simulink model "rfi_sim_model"  (R2013b)
settings: Solver=ode45  StartTime=0.0  StopTime=37888  RelTol=1e-3
undefined symbols (not defined in the file or in its folder): calan_lib, comp_addsub
libraries: xbsIndex_r4 x886, casper_library_misc x64, xps_library x1
(part 1 of 9)
settings Model: Creator=root  LastModifiedBy=root

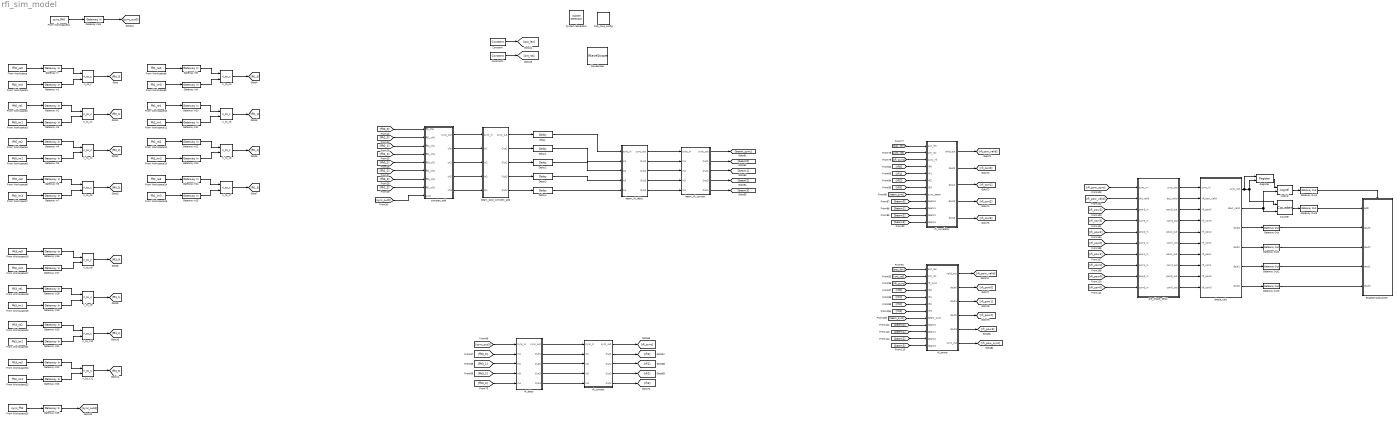
== system rfi_sim_model ==
  " System Generator" : xbsIndex_r4/ System Generator  Tag=genX  xilinxfamily=virtex6  part=xc6vsx475t  speed=-1  package=ff1759  synthesis_tool=XST  clock_wrapper=Clock Enables  directory=./arte/sysgen  proj_type=Project Navigator  Synth_file=XST Defaults  Impl_file=ISE Defaults  testbench=off  simulink_period=1  sysclk_period=6.6667  dcm_input_clock_period=100  incr_netlist=off  trim_vbits=Everywhere in SubSystem  dbl_ovrd=According to Block Masks  core_generation=According to Block Masks  run_coregen=off  deprecated_control=off  eval_field=0  block_type=sysgen
  Constant : xbsIndex_r4/Constant  const=64  gui_display_data_type=Fixed-point  arith_type=Unsigned  n_bits=16  bin_pt=0  preci_type=Single  exp_width=8  frac_width=24  explicit_period=on  period=1  equ=P=C  opselect=C  inp2=PCIN>>17  opr=+  inp1=P  carry=CIN  dbl_ovrd=off  block_type=constant
  Constant1 : xbsIndex_r4/Constant  const=0  gui_display_data_type=Boolean  arith_type=Boolean  n_bits=16  bin_pt=0  preci_type=Single  exp_width=8  frac_width=24  explicit_period=on  period=1  equ=P=C  opselect=C  inp2=PCIN>>17  opr=+  inp1=P  carry=CIN  dbl_ovrd=off  block_type=constant
  Counter : xbsIndex_r4/Counter  cnt_type=Free Running  cnt_to=Inf  operation=Up  start_count=0  cnt_by_val=1  arith_type=Unsigned  n_bits=9  bin_pt=0  load_pin=off  rst=on  en=on  explicit_period=on  period=1  dbl_ovrd=off  use_behavioral_HDL=off  implementation=Fabric  block_type=counter
  Delay{,1..4} (5 alike) : xbsIndex_r4/Delay  rst=off  infoeditControl=Selection of Reset will increase slice count due to use of real FFs and instead of SRLs  en=off  latency=1  dbl_ovrd=off  reg_retiming=off  block_type=delay
  Enabled Subsystem : Subsystem  TreatAsAtomicUnit=on
  From Workspace : FromWorkspace  VariableName=fft0_re0  SampleTime=1  Interpolate=off  OutputAfterFinalValue=Cyclic repetition
  From Workspace1 : FromWorkspace  VariableName=fft0_im0  SampleTime=1  Interpolate=off  OutputAfterFinalValue=Cyclic repetition
  From Workspace10 : FromWorkspace  VariableName=fft1_re1  SampleTime=1  Interpolate=off  OutputAfterFinalValue=Cyclic repetition
  From Workspace11 : FromWorkspace  VariableName=fft1_im1  SampleTime=1  Interpolate=off  OutputAfterFinalValue=Cyclic repetition
  From Workspace12 : FromWorkspace  VariableName=fft1_re2  SampleTime=1  Interpolate=off  OutputAfterFinalValue=Cyclic repetition
  From Workspace13 : FromWorkspace  VariableName=fft1_im2  SampleTime=1  Interpolate=off  OutputAfterFinalValue=Cyclic repetition
  From Workspace14 : FromWorkspace  VariableName=fft1_re3  SampleTime=1  Interpolate=off  OutputAfterFinalValue=Cyclic repetition
  From Workspace15 : FromWorkspace  VariableName=fft1_im3  SampleTime=1  Interpolate=off  OutputAfterFinalValue=Cyclic repetition
  From Workspace16 : FromWorkspace  VariableName=fft3_re0  SampleTime=1  Interpolate=off  OutputAfterFinalValue=Cyclic repetition
  From Workspace17 : FromWorkspace  VariableName=fft3_im0  SampleTime=1  Interpolate=off  OutputAfterFinalValue=Cyclic repetition
  From Workspace18 : FromWorkspace  VariableName=fft3_re1  SampleTime=1  Interpolate=off  OutputAfterFinalValue=Cyclic repetition
  From Workspace19 : FromWorkspace  VariableName=fft3_im1  SampleTime=1  Interpolate=off  OutputAfterFinalValue=Cyclic repetition
  From Workspace2 : FromWorkspace  VariableName=fft0_re1  SampleTime=1  Interpolate=off  OutputAfterFinalValue=Cyclic repetition
  From Workspace20 : FromWorkspace  VariableName=fft3_re2  SampleTime=1  Interpolate=off  OutputAfterFinalValue=Cyclic repetition
  From Workspace21 : FromWorkspace  VariableName=fft3_im2  SampleTime=1  Interpolate=off  OutputAfterFinalValue=Cyclic repetition
  From Workspace22 : FromWorkspace  VariableName=fft3_re3  SampleTime=1  Interpolate=off  OutputAfterFinalValue=Cyclic repetition
  From Workspace23 : FromWorkspace  VariableName=fft3_im3  SampleTime=1  Interpolate=off  OutputAfterFinalValue=Cyclic repetition
  From Workspace24 : FromWorkspace  VariableName=sync_fft0  SampleTime=1  Interpolate=off  OutputAfterFinalValue=Cyclic repetition
  From Workspace25 : FromWorkspace  VariableName=sync_fft3  SampleTime=1  Interpolate=off  OutputAfterFinalValue=Cyclic repetition
  From Workspace3 : FromWorkspace  VariableName=fft0_im1  SampleTime=1  Interpolate=off  OutputAfterFinalValue=Cyclic repetition
  From Workspace4 : FromWorkspace  VariableName=fft0_re2  SampleTime=1  Interpolate=off  OutputAfterFinalValue=Cyclic repetition
  From Workspace5 : FromWorkspace  VariableName=fft0_im2  SampleTime=1  Interpolate=off  OutputAfterFinalValue=Cyclic repetition
  From Workspace6 : FromWorkspace  VariableName=fft0_re3  SampleTime=1  Interpolate=off  OutputAfterFinalValue=Cyclic repetition
  From Workspace7 : FromWorkspace  VariableName=fft0_im3  SampleTime=1  Interpolate=off  OutputAfterFinalValue=Cyclic repetition
  From Workspace8 : FromWorkspace  VariableName=fft1_re0  SampleTime=1  Interpolate=off  OutputAfterFinalValue=Cyclic repetition
  From Workspace9 : FromWorkspace  VariableName=fft1_im0  SampleTime=1  Interpolate=off  OutputAfterFinalValue=Cyclic repetition
  Gateway In{,1..23} (24 alike) : xbsIndex_r4/Gateway In  gui_display_data_type=Fixed-point  arith_type="Signed  (2's comp)"  n_bits=18  bin_pt=17  preci_type=Single  exp_width=8  frac_width=24  quantization="Round  (unbiased: +/- Inf)"  overflow=Saturate  period=1  dbl_ovrd=off  timing_constraint=None  locs_specified=off  LOCs={}  UseAsADC=off  ADCChannel='1'  inherit_from_input=off  hdl_port=on  block_type=gatewayin
  Gateway In24 : xbsIndex_r4/Gateway In  gui_display_data_type=Boolean  arith_type=Boolean  n_bits=18  bin_pt=17  preci_type=Single  exp_width=8  frac_width=24  quantization="Round  (unbiased: +/- Inf)"  overflow=Saturate  period=1  dbl_ovrd=off  timing_constraint=None  locs_specified=off  LOCs={}  UseAsADC=off  ADCChannel='1'  inherit_from_input=off  hdl_port=on  block_type=gatewayin
  Gateway In25 : xbsIndex_r4/Gateway In  gui_display_data_type=Boolean  arith_type=Boolean  n_bits=18  bin_pt=17  preci_type=Single  exp_width=8  frac_width=24  quantization="Round  (unbiased: +/- Inf)"  overflow=Saturate  period=1  dbl_ovrd=off  timing_constraint=None  locs_specified=off  LOCs={}  UseAsADC=off  ADCChannel='1'  inherit_from_input=off  hdl_port=on  block_type=gatewayin
  Gateway Out{,1..5} (6 alike) : xbsIndex_r4/Gateway Out  inherit_from_input=off  hdl_port=on  timing_constraint=None  locs_specified=off  LOCs={}  UseAsDAC=off  DACChannel='1'  block_type=gatewayout
  Logical : xbsIndex_r4/Logical  logical_function=AND  inputs=2  en=off  latency=0  precision=Full  arith_type=Unsigned  n_bits=16  bin_pt=0  align_bp=on  dbl_ovrd=off  block_type=logical
  Register : xbsIndex_r4/Register  init=0  rst=off  en=on  dbl_ovrd=off  block_type=register
  WaveScope : xbsIndex_r4/WaveScope  block_type=wavescope
  XSG_core_config : xps_library/XSG_core_config  Tag=xps:xsg  hw_sys=ROACH2:sx475t  clk_src=adc0_clk  ROACH_clk_src=sys_clk  ROACH2_clk_src=adc0_clk  MKDIG_clk_src=sys_clk  clk_rate=150  sample_period=1  synthesis_tool=XST
  beam_post_complex_add : Subsystem  mask{lat=3}
  beam_rfi_convert : Subsystem  mask{shift_val=9, conv_width=9, conv_point=8}
      mask prompts: shift_val "shift"; conv_width "convert width"; conv_point "convert point"
  beam_rfi_delay : Subsystem  mask{lat=3}
  complex_add : Subsystem
  phase_calc : Subsystem  mask{din_width=16, din_point=2, scale_max_shift=10, scale_min_shift=3, pre_cordic_shift=0, pre_cordic_width=16, pre_cordic_point=2, cordic_iters=16}
      mask prompts: din_width "din width"; din_point "din point"; scale_max_shift "autoscale max shift"; scale_min_shift "autoscale min shift"; pre_cordic_shift "pre cordic shift"; pre_cordic_width "pre cordic width"; pre_cordic_point "pre cordic point"; cordic_iters "cordic iters"
  pre_phase_delay : Subsystem  mask{lat=2}
  rfi_convert : Subsystem  mask{shift_val=9, conv_width=9, conv_point=8}
      mask prompts: shift_val "shift"; conv_width "convert width"; conv_point "convert point"
  rfi_correlator : Subsystem  mask{din_width=9, din_point=8, cmult_width=18, cmult_point=16, cmult_add_dly=2, cmult_mult_dly=3, post_cmult_dly=1, acc_width=32, post_acc_dly=2, power_add_dly=2, power_mult_dly=3, dout_shift=11, dout_width=16, dout_point=2}
      mask prompts: din_width "din width"; din_point "din point"; cmult_width "cmult width"; cmult_point "cmult point"; cmult_add_dly "cmult add delay"; cmult_mult_dly "cmult mult delay"; post_cmult_dly "post cmult delay"; acc_width "acc width"; post_acc_dly "post acc delay"; power_add_dly "power add delay"; power_mult_dly "power mult delay"; dout_shift "output shift"; dout_width "output width"; dout_point "output point"
  rfi_delay : Subsystem  mask{lat=9}
  rfi_power : Subsystem  mask{din_width=9, din_point=8, pow_add_dly=2, pow_mult_dly=3, post_pow_dly=1, acc_width=32, post_acc_dly=2, post_acc_shift=0, post_acc_width=32, post_acc_point=16, cmult_add_dly=2, cmult_mult_dly=3, shift_out=11, dout_width=16, dout_point=2}
      mask prompts: din_width "din width"; pow_add_dly "power add delay"; pow_mult_dly "power mult delay"; post_pow_dly "post power delay"; acc_width "acc width"; post_acc_dly "post acc delay"; post_acc_shift "post acc shift"; post_acc_width "post acc width"; post_acc_point "post acc point"; cmult_add_dly "cmult add delay"; cmult_mult_dly "cmult mult delay"; shift_out "shift out"
  ri_to_c{,1..11} (12 alike) : casper_library_misc/ri_to_c
  wires:
  [fft0_0] -> complex_add/1(ff0_ch0)
  [fft1_0] -> complex_add/2(fft1_ch0)
  [fft0_1] -> complex_add/3(fft0_ch1)
  [fft1_1] -> complex_add/4(fft1_ch1)
  [fft0_2] -> complex_add/5(fft0_ch2)
  [fft1_2] -> complex_add/6(fft1_ch2)
  [fft0_3] -> complex_add/7(fft0_ch3)
  [fft1_3] -> complex_add/8(fft1_ch3)
  [sync_out0] -> complex_add/9(sync)
  complex_add/3(ch1) -> beam_post_complex_add/3(In2)
  complex_add/1(sync_out) -> beam_post_complex_add/1(sync_in)
  complex_add/2(ch0) -> beam_post_complex_add/2(In1)
  complex_add/5(ch3) -> beam_post_complex_add/5(In4)
  complex_add/4(ch2) -> beam_post_complex_add/4(In3)
  beam_post_complex_add/1(sync_out) -> Delay/1
  beam_post_complex_add/2(Out1) -> Delay1/1
  beam_post_complex_add/3(Out2) -> Delay2/1
  beam_post_complex_add/4(Out3) -> Delay3/1
  beam_post_complex_add/5(Out4) -> Delay4/1
  From Workspace/1 -> Gateway In/1
  From Workspace1/1 -> Gateway In1/1
  From Workspace2/1 -> Gateway In2/1
  From Workspace3/1 -> Gateway In3/1
  Gateway In/1 -> ri_to_c/1
  Gateway In1/1 -> ri_to_c/2
  Gateway In2/1 -> ri_to_c1/1
  Gateway In3/1 -> ri_to_c1/2
  From Workspace4/1 -> Gateway In4/1
  From Workspace5/1 -> Gateway In5/1
  From Workspace6/1 -> Gateway In6/1
  From Workspace7/1 -> Gateway In7/1
  Gateway In4/1 -> ri_to_c2/1
  Gateway In5/1 -> ri_to_c2/2
  Gateway In6/1 -> ri_to_c3/1
  Gateway In7/1 -> ri_to_c3/2
  ri_to_c/1 -> [fft0_0]
  ri_to_c1/1 -> [fft0_1]
  ri_to_c2/1 -> [fft0_2]
  ri_to_c3/1 -> [fft0_3]
  From Workspace8/1 -> Gateway In8/1
  From Workspace9/1 -> Gateway In9/1
  From Workspace10/1 -> Gateway In10/1
  From Workspace11/1 -> Gateway In11/1
  Gateway In8/1 -> ri_to_c4/1
  Gateway In9/1 -> ri_to_c4/2
  Gateway In10/1 -> ri_to_c5/1
  Gateway In11/1 -> ri_to_c5/2
  From Workspace12/1 -> Gateway In12/1
  From Workspace13/1 -> Gateway In13/1
  From Workspace14/1 -> Gateway In14/1
  From Workspace15/1 -> Gateway In15/1
  Gateway In12/1 -> ri_to_c6/1
  Gateway In13/1 -> ri_to_c6/2
  Gateway In14/1 -> ri_to_c7/1
  Gateway In15/1 -> ri_to_c7/2
  ri_to_c4/1 -> [fft1_0]
  ri_to_c5/1 -> [fft1_1]
  ri_to_c6/1 -> [fft1_2]
  ri_to_c7/1 -> [fft1_3]
  From Workspace16/1 -> Gateway In16/1
  From Workspace17/1 -> Gateway In17/1
  From Workspace18/1 -> Gateway In18/1
  From Workspace19/1 -> Gateway In19/1
  Gateway In16/1 -> ri_to_c8/1
  Gateway In17/1 -> ri_to_c8/2
  Gateway In18/1 -> ri_to_c9/1
  Gateway In19/1 -> ri_to_c9/2
  From Workspace20/1 -> Gateway In20/1
  From Workspace21/1 -> Gateway In21/1
  From Workspace22/1 -> Gateway In22/1
  From Workspace23/1 -> Gateway In23/1
  Gateway In20/1 -> ri_to_c10/1
  Gateway In21/1 -> ri_to_c10/2
  Gateway In22/1 -> ri_to_c11/1
  Gateway In23/1 -> ri_to_c11/2
  ri_to_c8/1 -> [fft3_0]
  ri_to_c9/1 -> [fft3_1]
  ri_to_c10/1 -> [fft3_2]
  ri_to_c11/1 -> [fft3_3]
  From Workspace24/1 -> Gateway In24/1
  Gateway In24/1 -> [sync_out0]
  From Workspace25/1 -> Gateway In25/1
  Gateway In25/1 -> [sync_out3]
  Delay/1 -> beam_rfi_delay/1(sync_in)
  Delay1/1 -> beam_rfi_delay/2(In1)
  Delay2/1 -> beam_rfi_delay/3(In2)
  Delay3/1 -> beam_rfi_delay/4(In3)
  Delay4/1 -> beam_rfi_delay/5(In4)
  Constant/1 -> [acc_len]
  Constant1/1 -> [cnt_rst]
  [acc_len] -> rfi_correlator/1(acc_len)
  [cnt_rst] -> rfi_correlator/2(cnt_rst)
  [rfi_sync] -> rfi_correlator/3(sync_rfi)
  [rfi0] -> rfi_correlator/4(rfi0)
  [rfi1] -> rfi_correlator/5(rfi1)
  [rfi2] -> rfi_correlator/6(rfi2)
  [rfi3] -> rfi_correlator/7(rfi3)
  [beam_sync] -> rfi_correlator/8(sync_beam)
  [beam0] -> rfi_correlator/9(beam0)
  [beam1] -> rfi_correlator/10(beam1)
  [beam2] -> rfi_correlator/11(beam2)
  [beam3] -> rfi_correlator/12(beam3)
  [acc_len] -> rfi_power/1(acc_len)
  [cnt_rst] -> rfi_power/2(cnt_rst)
  [rfi_sync] -> rfi_power/3(rfi_sync)
  [rfi0] -> rfi_power/4(rfi0)
  [rfi1] -> rfi_power/5(rfi1)
  [rfi2] -> rfi_power/6(rfi2)
  [rfi3] -> rfi_power/7(rfi3)
  [beam_sync] -> rfi_power/8(beam_sync)
  [beam0] -> rfi_power/9(beam0)
  [beam1] -> rfi_power/10(beam1)
  [beam2] -> rfi_power/11(beam2)
  [beam3] -> rfi_power/12(beam3)
  rfi_correlator/1(valid_out) -> [rfi_corr_valid]
  rfi_correlator/2(dout0) -> [rfi_corr0]
  rfi_correlator/3(dout1) -> [rfi_corr1]
  rfi_correlator/4(dout2) -> [rfi_corr2]
  rfi_correlator/5(dout3) -> [rfi_corr3]
  rfi_power/1(valid_out) -> [rfi_pow_valid]
  rfi_power/2(dout0) -> [rfi_pow0]
  rfi_power/3(dout1) -> [rfi_pow1]
  rfi_power/4(dout2) -> [rfi_pow2]
  rfi_power/5(dout3) -> [rfi_pow3]
  rfi_power/6(sync_out) -> [rfi_pow_sync]
  pre_phase_delay/3(pow3_out) -> phase_calc/3(rfi_pow3)
  pre_phase_delay/9(pow0_out) -> phase_calc/9(rfi_pow0)
  pre_phase_delay/5(pow2_out) -> phase_calc/5(rfi_pow2)
  pre_phase_delay/8(corr1_out) -> phase_calc/8(rfi_corr1)
  pre_phase_delay/1(sync_out) -> phase_calc/1(sync_in)
  pre_phase_delay/6(corr2_out) -> phase_calc/6(rfi_corr2)
  pre_phase_delay/10(corr0_out) -> phase_calc/10(rfi_corr0)
  pre_phase_delay/4(corr3_out) -> phase_calc/4(rfi_corr3)
  pre_phase_delay/7(pow1_out) -> phase_calc/7(rfi_pow1)
  pre_phase_delay/2(dou_valid) -> phase_calc/2(rfi_pow_valid)
  [rfi_pow_sync] -> pre_phase_delay/1(sync_in)
  [rfi_pow_valid] -> pre_phase_delay/2(din_valid)
  [rfi_pow3] -> pre_phase_delay/3(pow3_in)
  [rfi_corr3] -> pre_phase_delay/4(corr3_in)
  [rfi_pow2] -> pre_phase_delay/5(pow2_in)
  [rfi_corr2] -> pre_phase_delay/6(corr2_in)
  [rfi_pow1] -> pre_phase_delay/7(pow1_in)
  [rfi_corr1] -> pre_phase_delay/8(corr1_in)
  [rfi_pow0] -> pre_phase_delay/9(pow0_in)
  [rfi_corr0] -> pre_phase_delay/10(corr0_in)
  rfi_delay/2(Out1) -> rfi_convert/2(In1)
  rfi_delay/3(Out2) -> rfi_convert/3(In2)
  rfi_delay/1(sync_out) -> rfi_convert/1(sync_in)
  rfi_delay/4(Out3) -> rfi_convert/4(In3)
  rfi_delay/5(Out4) -> rfi_convert/5(In4)
  [sync_out3] -> rfi_delay/1(sync_in)
  [fft3_0] -> rfi_delay/2(In1)
  [fft3_1] -> rfi_delay/3(In2)
  [fft3_2] -> rfi_delay/4(In3)
  [fft3_3] -> rfi_delay/5(In4)
  rfi_convert/1(sync_out) -> [rfi_sync]
  rfi_convert/2(Out1) -> [rfi0]
  rfi_convert/3(Out2) -> [rfi1]
  rfi_convert/4(Out3) -> [rfi2]
  rfi_convert/5(Out4) -> [rfi3]
  beam_rfi_delay/2(Out1) -> beam_rfi_convert/2(In1)
  beam_rfi_delay/3(Out2) -> beam_rfi_convert/3(In2)
  beam_rfi_delay/1(sync_out) -> beam_rfi_convert/1(sync_in)
  beam_rfi_delay/4(Out3) -> beam_rfi_convert/4(In3)
  beam_rfi_delay/5(Out4) -> beam_rfi_convert/5(In4)
  beam_rfi_convert/1(sync_out) -> [beam_sync]
  beam_rfi_convert/2(Out1) -> [beam0]
  beam_rfi_convert/3(Out2) -> [beam1]
  beam_rfi_convert/4(Out3) -> [beam2]
  beam_rfi_convert/5(Out4) -> [beam3]
  phase_calc/3(dout3) -> Gateway Out/1
  phase_calc/4(dout2) -> Gateway Out1/1
  phase_calc/5(dout1) -> Gateway Out2/1
  phase_calc/6(dout0) -> Gateway Out3/1
  phase_calc/1(sync_out) -> Register/1, Counter/1, Register/2
  phase_calc/2(dout_valid) -> Logical/2, Counter/2
  Register/1 -> Logical/1
  Logical/1 -> Gateway Out4/1
  Gateway Out4/1 -> Enabled Subsystem/Enable
  Gateway Out/1 -> Enabled Subsystem/2(dout3)
  Gateway Out1/1 -> Enabled Subsystem/3(dout2)
  Gateway Out2/1 -> Enabled Subsystem/4(dout1)
  Gateway Out3/1 -> Enabled Subsystem/5(dout0)
  Counter/1 -> Gateway Out5/1
  Gateway Out5/1 -> Enabled Subsystem/1(addr)

== system rfi_sim_model/Enabled Subsystem ==
  addr : Inport
  dout3 : Inport  Port=2
  dout2 : Inport  Port=3
  dout1 : Inport  Port=4
  dout0 : Inport  Port=5
  Enable : EnablePort
  To Workspace : ToWorkspace  VariableName=dout3  SampleTime=-1  SaveFormat=Timeseries
  To Workspace1 : ToWorkspace  VariableName=dout2  SampleTime=-1  SaveFormat=Timeseries
  To Workspace2 : ToWorkspace  VariableName=dout1  SampleTime=-1  SaveFormat=Timeseries
  To Workspace3 : ToWorkspace  VariableName=dout0  SampleTime=-1  SaveFormat=Timeseries
  To Workspace4 : ToWorkspace  VariableName=addr  SampleTime=-1  SaveFormat=Timeseries
  wires:
  dout3/1 -> To Workspace/1
  dout2/1 -> To Workspace1/1
  dout1/1 -> To Workspace2/1
  dout0/1 -> To Workspace3/1
  addr/1 -> To Workspace4/1

== system rfi_sim_model/beam_post_complex_add ==
  sync_in : Inport
  In1 : Inport  Port=2
  In2 : Inport  Port=3
  In3 : Inport  Port=4
  In4 : Inport  Port=5
  pipeline1 : Subsystem  AncestorBlock=casper_library_delays/pipeline  mask(pipeline){latency=lat}
      mask help:
      | An explicitly laid-out delay line to avoid mapping to SRL16s
      | for use in pipelining to help achieve timing closure.
      mask init:
      | pipeline_init(gcb,'latency',latency);
      settings: AttributesFormatString=Latency = %<latency>
      mask Display:
      | port_label('input', 1, 'd');
      | port_label('output', 1, 'q');
      | disp(['Z^-', num2str(latency)]);
  pipeline2 : Subsystem  AncestorBlock=casper_library_delays/pipeline  mask(pipeline){latency=lat}
      mask help:
      | An explicitly laid-out delay line to avoid mapping to SRL16s
      | for use in pipelining to help achieve timing closure.
      mask init:
      | pipeline_init(gcb,'latency',latency);
      settings: AttributesFormatString=Latency = %<latency>
      mask Display:
      | port_label('input', 1, 'd');
      | port_label('output', 1, 'q');
      | disp(['Z^-', num2str(latency)]);
  pipeline3 : Subsystem  AncestorBlock=casper_library_delays/pipeline  mask(pipeline){latency=lat}
      mask help:
      | An explicitly laid-out delay line to avoid mapping to SRL16s
      | for use in pipelining to help achieve timing closure.
      mask init:
      | pipeline_init(gcb,'latency',latency);
      settings: AttributesFormatString=Latency = %<latency>
      mask Display:
      | port_label('input', 1, 'd');
      | port_label('output', 1, 'q');
      | disp(['Z^-', num2str(latency)]);
  pipeline4 : Subsystem  AncestorBlock=casper_library_delays/pipeline  mask(pipeline){latency=lat}
      mask help:
      | An explicitly laid-out delay line to avoid mapping to SRL16s
      | for use in pipelining to help achieve timing closure.
      mask init:
      | pipeline_init(gcb,'latency',latency);
      settings: AttributesFormatString=Latency = %<latency>
      mask Display:
      | port_label('input', 1, 'd');
      | port_label('output', 1, 'q');
      | disp(['Z^-', num2str(latency)]);
  pipeline5 : Subsystem  AncestorBlock=casper_library_delays/pipeline  mask(pipeline){latency=lat}
      mask help:
      | An explicitly laid-out delay line to avoid mapping to SRL16s
      | for use in pipelining to help achieve timing closure.
      mask init:
      | pipeline_init(gcb,'latency',latency);
      settings: AttributesFormatString=Latency = %<latency>
      mask Display:
      | port_label('input', 1, 'd');
      | port_label('output', 1, 'q');
      | disp(['Z^-', num2str(latency)]);
  sync_out : Outport
  Out1 : Outport  Port=2
  Out2 : Outport  Port=3
  Out3 : Outport  Port=4
  Out4 : Outport  Port=5
  wires:
  sync_in/1 -> pipeline1/1(d)
  pipeline1/1(q) -> sync_out/1
  In1/1 -> pipeline2/1(d)
  pipeline2/1(q) -> Out1/1
  In2/1 -> pipeline3/1(d)
  pipeline3/1(q) -> Out2/1
  In3/1 -> pipeline4/1(d)
  pipeline4/1(q) -> Out3/1
  In4/1 -> pipeline5/1(d)
  pipeline5/1(q) -> Out4/1

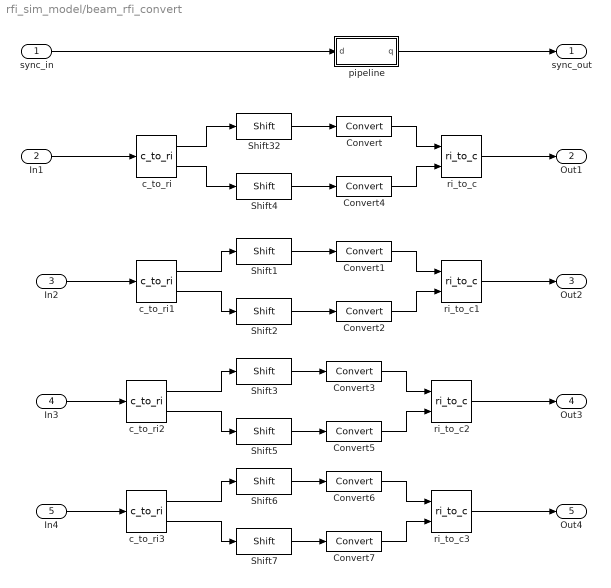
== system rfi_sim_model/beam_rfi_convert ==
  sync_in : Inport
  In1 : Inport  Port=2
  In2 : Inport  Port=3
  In3 : Inport  Port=4
  In4 : Inport  Port=5
  Convert{,1..7} (8 alike) : xbsIndex_r4/Convert  gui_display_data_type=Fixed-point  arith_type="Signed  (2's comp)"  n_bits=conv_width  bin_pt=conv_point  float_type=Single  exp_bits=8  fraction_bits=24  quantization=Truncate  overflow=Wrap  en=off  latency=2  dbl_ovrd=off  pipeline=off  block_type=convert
      settings: block_version=11.4
  Shift{1..7,32} (8 alike) : xbsIndex_r4/Shift  shift_dir=Left  shift_bits=shift_val  en=off  latency=0  precision=Full  arith_type="Signed  (2's comp)"  n_bits=16  bin_pt=14  quantization=Truncate  overflow=Wrap  dbl_ovrd=off  block_type=shift
  c_to_ri{,1..3} (4 alike) : casper_library_misc/c_to_ri  n_bits=18  bin_pt=17
  pipeline : Subsystem  AncestorBlock=casper_library_delays/pipeline  mask(pipeline){latency=2}
      mask help:
      | An explicitly laid-out delay line to avoid mapping to SRL16s
      | for use in pipelining to help achieve timing closure.
      mask init:
      | pipeline_init(gcb,'latency',latency);
      settings: AttributesFormatString=Latency = %<latency>
      mask Display:
      | port_label('input', 1, 'd');
      | port_label('output', 1, 'q');
      | disp(['Z^-', num2str(latency)]);
  ri_to_c{,1..3} (4 alike) : casper_library_misc/ri_to_c
  sync_out : Outport
  Out1 : Outport  Port=2
  Out2 : Outport  Port=3
  Out3 : Outport  Port=4
  Out4 : Outport  Port=5
  wires:
  Shift32/1 -> Convert/1
  sync_in/1 -> pipeline/1(d)
  pipeline/1(q) -> sync_out/1
  In1/1 -> c_to_ri/1
  c_to_ri/1 -> Shift32/1
  ri_to_c/1 -> Out1/1
  Convert/1 -> ri_to_c/1
  Shift4/1 -> Convert4/1
  c_to_ri/2 -> Shift4/1
  Convert4/1 -> ri_to_c/2
  Shift1/1 -> Convert1/1
  c_to_ri1/1 -> Shift1/1
  ri_to_c1/1 -> Out2/1
  Convert1/1 -> ri_to_c1/1
  Shift2/1 -> Convert2/1
  c_to_ri1/2 -> Shift2/1
  Convert2/1 -> ri_to_c1/2
  In2/1 -> c_to_ri1/1
  Shift3/1 -> Convert3/1
  c_to_ri2/1 -> Shift3/1
  ri_to_c2/1 -> Out3/1
  Convert3/1 -> ri_to_c2/1
  Shift5/1 -> Convert5/1
  c_to_ri2/2 -> Shift5/1
  Convert5/1 -> ri_to_c2/2
  In3/1 -> c_to_ri2/1
  Shift6/1 -> Convert6/1
  c_to_ri3/1 -> Shift6/1
  ri_to_c3/1 -> Out4/1
  Convert6/1 -> ri_to_c3/1
  Shift7/1 -> Convert7/1
  c_to_ri3/2 -> Shift7/1
  Convert7/1 -> ri_to_c3/2
  In4/1 -> c_to_ri3/1

== system rfi_sim_model/beam_rfi_delay ==
  sync_in : Inport
  In1 : Inport  Port=2
  In2 : Inport  Port=3
  In3 : Inport  Port=4
  In4 : Inport  Port=5
  pipeline1 : Subsystem  AncestorBlock=casper_library_delays/pipeline  mask(pipeline){latency=lat}
      mask help:
      | An explicitly laid-out delay line to avoid mapping to SRL16s
      | for use in pipelining to help achieve timing closure.
      mask init:
      | pipeline_init(gcb,'latency',latency);
      settings: AttributesFormatString=Latency = %<latency>
      mask Display:
      | port_label('input', 1, 'd');
      | port_label('output', 1, 'q');
      | disp(['Z^-', num2str(latency)]);
  pipeline2 : Subsystem  AncestorBlock=casper_library_delays/pipeline  mask(pipeline){latency=lat}
      mask help:
      | An explicitly laid-out delay line to avoid mapping to SRL16s
      | for use in pipelining to help achieve timing closure.
      mask init:
      | pipeline_init(gcb,'latency',latency);
      settings: AttributesFormatString=Latency = %<latency>
      mask Display:
      | port_label('input', 1, 'd');
      | port_label('output', 1, 'q');
      | disp(['Z^-', num2str(latency)]);
  pipeline3 : Subsystem  AncestorBlock=casper_library_delays/pipeline  mask(pipeline){latency=lat}
      mask help:
      | An explicitly laid-out delay line to avoid mapping to SRL16s
      | for use in pipelining to help achieve timing closure.
      mask init:
      | pipeline_init(gcb,'latency',latency);
      settings: AttributesFormatString=Latency = %<latency>
      mask Display:
      | port_label('input', 1, 'd');
      | port_label('output', 1, 'q');
      | disp(['Z^-', num2str(latency)]);
  pipeline4 : Subsystem  AncestorBlock=casper_library_delays/pipeline  mask(pipeline){latency=lat}
      mask help:
      | An explicitly laid-out delay line to avoid mapping to SRL16s
      | for use in pipelining to help achieve timing closure.
      mask init:
      | pipeline_init(gcb,'latency',latency);
      settings: AttributesFormatString=Latency = %<latency>
      mask Display:
      | port_label('input', 1, 'd');
      | port_label('output', 1, 'q');
      | disp(['Z^-', num2str(latency)]);
  pipeline5 : Subsystem  AncestorBlock=casper_library_delays/pipeline  mask(pipeline){latency=lat}
      mask help:
      | An explicitly laid-out delay line to avoid mapping to SRL16s
      | for use in pipelining to help achieve timing closure.
      mask init:
      | pipeline_init(gcb,'latency',latency);
      settings: AttributesFormatString=Latency = %<latency>
      mask Display:
      | port_label('input', 1, 'd');
      | port_label('output', 1, 'q');
      | disp(['Z^-', num2str(latency)]);
  sync_out : Outport
  Out1 : Outport  Port=2
  Out2 : Outport  Port=3
  Out3 : Outport  Port=4
  Out4 : Outport  Port=5
  wires:
  sync_in/1 -> pipeline1/1(d)
  pipeline1/1(q) -> sync_out/1
  In1/1 -> pipeline2/1(d)
  pipeline2/1(q) -> Out1/1
  In2/1 -> pipeline3/1(d)
  pipeline3/1(q) -> Out2/1
  In3/1 -> pipeline4/1(d)
  pipeline4/1(q) -> Out3/1
  In4/1 -> pipeline5/1(d)
  pipeline5/1(q) -> Out4/1

== system rfi_sim_model/complex_add ==
  ff0_ch0 : Inport
  fft1_ch0 : Inport  Port=2
  fft0_ch1 : Inport  Port=3
  fft1_ch1 : Inport  Port=4
  fft0_ch2 : Inport  Port=5
  fft1_ch2 : Inport  Port=6
  fft0_ch3 : Inport  Port=7
  fft1_ch3 : Inport  Port=8
  sync : Inport  Port=9
  comp_addsub : Subsystem  AncestorBlock=calan_lib/comp_addsub  mask(comp_addsub){addsub=Addition, n_bits_in=18, bin_pt_in=17, add_latency=2, n_bits_out=18, bin_pt_out=17, quantization=Truncate, overflow=Wrap}
      mask prompts: addsub "Addition/Subtraction"; n_bits_in "Bit Width"; bin_pt_in "Binary Point"; add_latency "Adder Latency"; n_bits_out "Bit Width"; bin_pt_out "BInary Point"
      mask help: Add or substract two complex numbers of the same length.
      mask init:
      | comp_addsub_init(gcb, ...
      |     'addsub', addsub, ...
      |     'n_bits_in', n_bits_in, ...
      |     'bin_pt_in', bin_pt_in, ...
      |     'n_bits_out', n_bits_out, ...
      |     'bin_pt_out', bin_pt_out, ...
      |     'quantization', quantization, ...
      |     'overflow', overflow, ...
      |     'add_latency', add_latency);
      settings: AttributesFormatString=|
      | 18_17 * 18_17 ==> 18_17
      | Truncate, Wrap
      mask TypeOptions addsub: Addition | Subtraction
      mask TypeOptions quantization: Truncate | Round  (unbiased: +/- Inf)
      mask TypeOptions overflow: Wrap | Saturate | Flag as error
      mask Display:
      | port_label('input', 1, 'a');
      | port_label('input', 2, 'b');
      | if strcmp(addsub, 'Addition')
      |     port_label('output', 1, 'a+b');
      | elseif strcmp(addsub, 'Subtraction')
      |     port_label('output', 1, 'a-b');
      | end
      | disp(['Z^-', num2str(add_latency)]);
  comp_addsub1 : Subsystem  AncestorBlock=calan_lib/comp_addsub  mask(comp_addsub){addsub=Addition, n_bits_in=18, bin_pt_in=17, add_latency=2, n_bits_out=18, bin_pt_out=17, quantization=Truncate, overflow=Wrap}
      mask prompts: addsub "Addition/Subtraction"; n_bits_in "Bit Width"; bin_pt_in "Binary Point"; add_latency "Adder Latency"; n_bits_out "Bit Width"; bin_pt_out "BInary Point"
      mask help: Add or substract two complex numbers of the same length.
      mask init: same as rfi_sim_model/complex_add/comp_addsub
      settings: AttributesFormatString=|
      | 18_17 * 18_17 ==> 18_17
      | Truncate, Wrap
      mask TypeOptions addsub: Addition | Subtraction
      mask TypeOptions quantization: Truncate | Round  (unbiased: +/- Inf)
      mask TypeOptions overflow: Wrap | Saturate | Flag as error
      mask Display:
      | port_label('input', 1, 'a');
      | port_label('input', 2, 'b');
      | if strcmp(addsub, 'Addition')
      |     port_label('output', 1, 'a+b');
      | elseif strcmp(addsub, 'Subtraction')
      |     port_label('output', 1, 'a-b');
      | end
      | disp(['Z^-', num2str(add_latency)]);
  comp_addsub3 : Subsystem  AncestorBlock=calan_lib/comp_addsub  mask(comp_addsub){addsub=Addition, n_bits_in=18, bin_pt_in=17, add_latency=2, n_bits_out=18, bin_pt_out=17, quantization=Truncate, overflow=Wrap}
      mask prompts: addsub "Addition/Subtraction"; n_bits_in "Bit Width"; bin_pt_in "Binary Point"; add_latency "Adder Latency"; n_bits_out "Bit Width"; bin_pt_out "BInary Point"
      mask help: Add or substract two complex numbers of the same length.
      mask init: same as rfi_sim_model/complex_add/comp_addsub
      settings: AttributesFormatString=|
      | 18_17 * 18_17 ==> 18_17
      | Truncate, Wrap
      mask TypeOptions addsub: Addition | Subtraction
      mask TypeOptions quantization: Truncate | Round  (unbiased: +/- Inf)
      mask TypeOptions overflow: Wrap | Saturate | Flag as error
      mask Display:
      | port_label('input', 1, 'a');
      | port_label('input', 2, 'b');
      | if strcmp(addsub, 'Addition')
      |     port_label('output', 1, 'a+b');
      | elseif strcmp(addsub, 'Subtraction')
      |     port_label('output', 1, 'a-b');
      | end
      | disp(['Z^-', num2str(add_latency)]);
  comp_addsub6 : Subsystem  AncestorBlock=calan_lib/comp_addsub  mask(comp_addsub){addsub=Addition, n_bits_in=18, bin_pt_in=17, add_latency=2, n_bits_out=18, bin_pt_out=17, quantization=Truncate, overflow=Wrap}
      mask prompts: addsub "Addition/Subtraction"; n_bits_in "Bit Width"; bin_pt_in "Binary Point"; add_latency "Adder Latency"; n_bits_out "Bit Width"; bin_pt_out "BInary Point"
      mask help: Add or substract two complex numbers of the same length.
      mask init: same as rfi_sim_model/complex_add/comp_addsub
      settings: AttributesFormatString=|
      | 18_17 * 18_17 ==> 18_17
      | Truncate, Wrap
      mask TypeOptions addsub: Addition | Subtraction
      mask TypeOptions quantization: Truncate | Round  (unbiased: +/- Inf)
      mask TypeOptions overflow: Wrap | Saturate | Flag as error
      mask Display:
      | port_label('input', 1, 'a');
      | port_label('input', 2, 'b');
      | if strcmp(addsub, 'Addition')
      |     port_label('output', 1, 'a+b');
      | elseif strcmp(addsub, 'Subtraction')
      |     port_label('output', 1, 'a-b');
      | end
      | disp(['Z^-', num2str(add_latency)]);
  pipeline4 : Subsystem  AncestorBlock=casper_library_delays/pipeline  mask(pipeline){latency=2}
      mask help:
      | An explicitly laid-out delay line to avoid mapping to SRL16s
      | for use in pipelining to help achieve timing closure.
      mask init:
      | pipeline_init(gcb,'latency',latency);
      settings: AttributesFormatString=Latency = %<latency>
      mask Display:
      | port_label('input', 1, 'd');
      | port_label('output', 1, 'q');
      | disp(['Z^-', num2str(latency)]);
  sync_out : Outport
  ch0 : Outport  Port=2
  ch1 : Outport  Port=3
  ch2 : Outport  Port=4
  ch3 : Outport  Port=5
  wires:
  ff0_ch0/1 -> comp_addsub/1(a)
  fft1_ch0/1 -> comp_addsub/2(b)
  fft0_ch1/1 -> comp_addsub1/1(a)
  fft1_ch1/1 -> comp_addsub1/2(b)
  fft0_ch2/1 -> comp_addsub3/1(a)
  comp_addsub3/1(out) -> ch2/1
  fft1_ch2/1 -> comp_addsub3/2(b)
  fft0_ch3/1 -> comp_addsub6/1(a)
  fft1_ch3/1 -> comp_addsub6/2(b)
  sync/1 -> pipeline4/1(d)
  pipeline4/1(q) -> sync_out/1
  comp_addsub/1(out) -> ch0/1
  comp_addsub6/1(out) -> ch3/1
  comp_addsub1/1(out) -> ch1/1

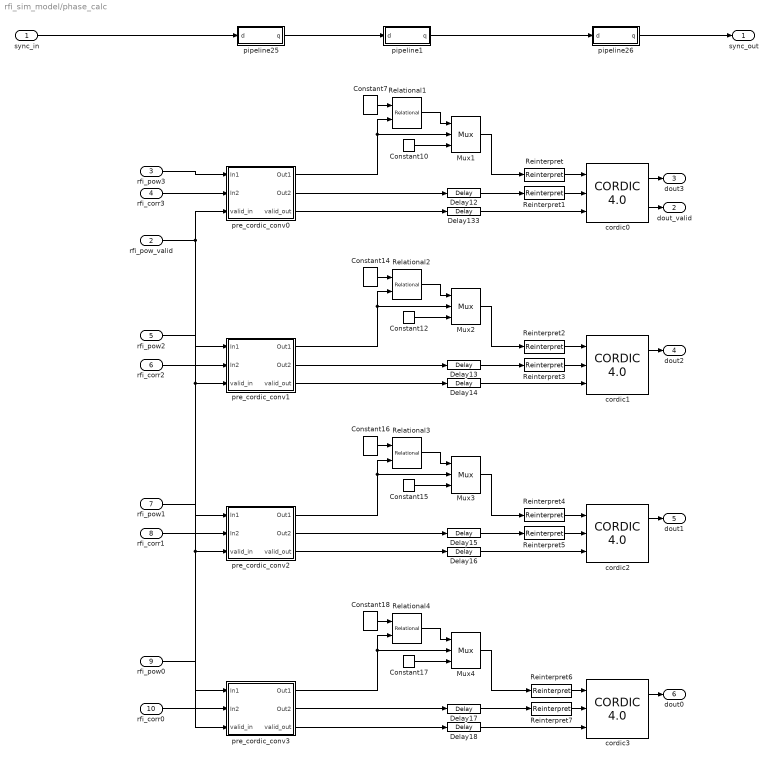
== system rfi_sim_model/phase_calc ==
  sync_in : Inport
  rfi_pow_valid : Inport  Port=2
  rfi_pow3 : Inport  Port=3
  rfi_corr3 : Inport  Port=4
  rfi_pow2 : Inport  Port=5
  rfi_corr2 : Inport  Port=6
  rfi_pow1 : Inport  Port=7
  rfi_corr1 : Inport  Port=8
  rfi_pow0 : Inport  Port=9
  rfi_corr0 : Inport  Port=10
  Constant{10,12,15,17} (4 alike) : xbsIndex_r4/Constant  const=1  gui_display_data_type=Fixed-point  arith_type=Signed (2's comp)  n_bits=pre_cordic_width  bin_pt=pre_cordic_point  preci_type=Single  exp_width=8  frac_width=24  explicit_period=on  period=1  equ=P=C  opselect=C  inp2=PCIN>>17  opr=+  inp1=P  carry=CIN  dbl_ovrd=off  block_type=constant
  Constant{7,14,16,18} (4 alike) : xbsIndex_r4/Constant  const=0  gui_display_data_type=Fixed-point  arith_type=Signed (2's comp)  n_bits=pre_cordic_width  bin_pt=pre_cordic_point  preci_type=Single  exp_width=8  frac_width=24  explicit_period=on  period=1  equ=P=C  opselect=C  inp2=PCIN>>17  opr=+  inp1=P  carry=CIN  dbl_ovrd=off  block_type=constant
  Delay{12..18,133} (8 alike) : xbsIndex_r4/Delay  rst=off  infoeditControl=Selection of Reset will increase slice count due to use of real FFs and instead of SRLs  en=off  latency=1  dbl_ovrd=off  reg_retiming=off  block_type=delay
  Mux{1..4} (4 alike) : xbsIndex_r4/Mux  inputs=2  en=off  latency=1  precision=Full  arith_type=Unsigned  n_bits=16  bin_pt=14  quantization=Truncate  overflow=Wrap  dbl_ovrd=off  block_type=mux
  Reinterpret{,1..7} (8 alike) : xbsIndex_r4/Reinterpret  force_arith_type=off  arith_type=Unsigned  force_bin_pt=on  bin_pt=pre_cordic_width-2  block_type=reinterpret
  Relational{1..4} (4 alike) : xbsIndex_r4/Relational  mode=a=b  en=off  latency=0  dbl_ovrd=off  block_type=relational
  cordic{0..3} (4 alike) : xbsIndex_r4/CORDIC 4.0   functional_selection=Arc_Tan  architectural_configuration=Parallel  pipelining_mode=Maximum  data_format=SignedFraction  phase_format=Radians  output_width=cordic_iters  round_mode=Truncate  iterations=cordic_iters  precision=0  coarse_rotation=off  compensation_scaling=No_Scale_Compensation  ce=off  sclr=off  nd=on  rdy=on  x_out=off  y_out=off  phase_output=on  register_inputs=true  register_outputs=true  ipcore_usecache=true  ipcore_useipmodelcache=true  ipcore_verbose=false  wrapper_available=true  ip_name=CORDIC  ip_version=4.0  dsptool_ready=true  port_translation_map={ 'ce' => 'en', 'sclr' => 'rst' }  structural_sim=false  block_type=cordic_v4_0
  pipeline1 : Subsystem  AncestorBlock=casper_library_delays/pipeline  mask(pipeline){latency=1}
      mask help:
      | An explicitly laid-out delay line to avoid mapping to SRL16s
      | for use in pipelining to help achieve timing closure.
      mask init:
      | pipeline_init(gcb,'latency',latency);
      settings: AttributesFormatString=Latency = %<latency>
      mask Display:
      | port_label('input', 1, 'd');
      | port_label('output', 1, 'q');
      | disp(['Z^-', num2str(latency)]);
  pipeline25 : Subsystem  AncestorBlock=casper_library_delays/pipeline  mask(pipeline){latency=2}
      mask help:
      | An explicitly laid-out delay line to avoid mapping to SRL16s
      | for use in pipelining to help achieve timing closure.
      mask init:
      | pipeline_init(gcb,'latency',latency);
      settings: AttributesFormatString=Latency = %<latency>
      mask Display:
      | port_label('input', 1, 'd');
      | port_label('output', 1, 'q');
      | disp(['Z^-', num2str(latency)]);
  pipeline26 : Subsystem  AncestorBlock=casper_library_delays/pipeline  mask(pipeline){latency=cordic_iters+2}
      mask help:
      | An explicitly laid-out delay line to avoid mapping to SRL16s
      | for use in pipelining to help achieve timing closure.
      mask init:
      | pipeline_init(gcb,'latency',latency);
      settings: AttributesFormatString=Latency = %<latency>
      mask Display:
      | port_label('input', 1, 'd');
      | port_label('output', 1, 'q');
      | disp(['Z^-', num2str(latency)]);
  pre_cordic_conv0 : Subsystem  mask{shift_val=pre_cordic_shift, conv_width=pre_cordic_width, conv_point=pre_cordic_point}
      mask prompts: shift_val "shift"; conv_width "convert width"; conv_point "convert point"
  pre_cordic_conv1 : Subsystem  mask{shift_val=pre_cordic_shift, conv_width=pre_cordic_width, conv_point=pre_cordic_point}
      mask prompts: shift_val "shift"; conv_width "convert width"; conv_point "convert point"
  pre_cordic_conv2 : Subsystem  mask{shift_val=pre_cordic_shift, conv_width=pre_cordic_width, conv_point=pre_cordic_point}
      mask prompts: shift_val "shift"; conv_width "convert width"; conv_point "convert point"
  pre_cordic_conv3 : Subsystem  mask{shift_val=pre_cordic_shift, conv_width=pre_cordic_width, conv_point=pre_cordic_point}
      mask prompts: shift_val "shift"; conv_width "convert width"; conv_point "convert point"
  sync_out : Outport
  dout_valid : Outport  Port=2
  dout3 : Outport  Port=3
  dout2 : Outport  Port=4
  dout1 : Outport  Port=5
  dout0 : Outport  Port=6
  wires:
  rfi_pow1/1 -> pre_cordic_conv2/1(In1)
  Delay14/1 -> cordic1/3
  pre_cordic_conv2/2(Out2) -> Delay15/1
  Mux3/1 -> Reinterpret4/1
  cordic1/1 -> dout2/1
  pipeline26/1(q) -> sync_out/1
  Delay13/1 -> Reinterpret3/1
  pre_cordic_conv1/2(Out2) -> Delay13/1
  Mux2/1 -> Reinterpret2/1
  pre_cordic_conv1/3(valid_out) -> Delay14/1
  Constant15/1 -> Mux3/3
  Delay15/1 -> Reinterpret5/1
  cordic0/2 -> dout_valid/1
  Constant16/1 -> Relational3/1
  rfi_corr1/1 -> pre_cordic_conv2/2(In2)
  rfi_pow0/1 -> pre_cordic_conv3/1(In1)
  rfi_corr0/1 -> pre_cordic_conv3/2(In2)
  rfi_pow_valid/1 -> pre_cordic_conv0/3(valid_in), pre_cordic_conv3/3(valid_in), pre_cordic_conv2/3(valid_in), pre_cordic_conv1/3(valid_in)
  pre_cordic_conv3/1(Out1) -> Mux4/2, Relational4/2
  Relational4/1 -> Mux4/1
  Constant18/1 -> Relational4/1
  Constant17/1 -> Mux4/3
  Delay17/1 -> Reinterpret7/1
  pre_cordic_conv3/2(Out2) -> Delay17/1
  Mux4/1 -> Reinterpret6/1
  pre_cordic_conv3/3(valid_out) -> Delay18/1
  Delay18/1 -> cordic3/3
  cordic2/1 -> dout1/1
  pre_cordic_conv0/1(Out1) -> Mux1/2, Relational1/2
  rfi_corr2/1 -> pre_cordic_conv1/2(In2)
  pre_cordic_conv1/1(Out1) -> Mux2/2, Relational2/2
  Constant10/1 -> Mux1/3
  rfi_pow3/1 -> pre_cordic_conv0/1(In1)
  sync_in/1 -> pipeline25/1(d)
  pre_cordic_conv0/3(valid_out) -> Delay133/1
  Mux1/1 -> Reinterpret/1
  Constant7/1 -> Relational1/1
  Delay133/1 -> cordic0/3
  pre_cordic_conv0/2(Out2) -> Delay12/1
  cordic0/1 -> dout3/1
  cordic3/1 -> dout0/1
  pre_cordic_conv2/1(Out1) -> Mux3/2, Relational3/2
  Relational3/1 -> Mux3/1
  rfi_corr3/1 -> pre_cordic_conv0/2(In2)
  pipeline25/1(q) -> pipeline1/1(d)
  Relational1/1 -> Mux1/1
  rfi_pow2/1 -> pre_cordic_conv1/1(In1)
  Delay12/1 -> Reinterpret1/1
  pre_cordic_conv2/3(valid_out) -> Delay16/1
  Delay16/1 -> cordic2/3
  Relational2/1 -> Mux2/1
  Constant14/1 -> Relational2/1
  Constant12/1 -> Mux2/3
  Reinterpret/1 -> cordic0/1
  Reinterpret1/1 -> cordic0/2
  Reinterpret3/1 -> cordic1/2
  Reinterpret2/1 -> cordic1/1
  Reinterpret4/1 -> cordic2/1
  Reinterpret5/1 -> cordic2/2
  Reinterpret6/1 -> cordic3/1
  Reinterpret7/1 -> cordic3/2
  pipeline1/1(q) -> pipeline26/1(d)

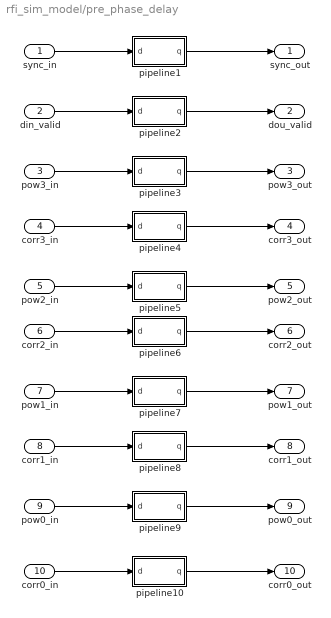
== system rfi_sim_model/pre_phase_delay ==
  sync_in : Inport
  din_valid : Inport  Port=2
  pow3_in : Inport  Port=3
  corr3_in : Inport  Port=4
  pow2_in : Inport  Port=5
  corr2_in : Inport  Port=6
  pow1_in : Inport  Port=7
  corr1_in : Inport  Port=8
  pow0_in : Inport  Port=9
  corr0_in : Inport  Port=10
  pipeline1 : Subsystem  AncestorBlock=casper_library_delays/pipeline  mask(pipeline){latency=lat}
      mask help:
      | An explicitly laid-out delay line to avoid mapping to SRL16s
      | for use in pipelining to help achieve timing closure.
      mask init:
      | pipeline_init(gcb,'latency',latency);
      settings: AttributesFormatString=Latency = %<latency>
      mask Display:
      | port_label('input', 1, 'd');
      | port_label('output', 1, 'q');
      | disp(['Z^-', num2str(latency)]);
  pipeline10 : Subsystem  AncestorBlock=casper_library_delays/pipeline  mask(pipeline){latency=lat}
      mask help:
      | An explicitly laid-out delay line to avoid mapping to SRL16s
      | for use in pipelining to help achieve timing closure.
      mask init:
      | pipeline_init(gcb,'latency',latency);
      settings: AttributesFormatString=Latency = %<latency>
      mask Display:
      | port_label('input', 1, 'd');
      | port_label('output', 1, 'q');
      | disp(['Z^-', num2str(latency)]);
  pipeline2 : Subsystem  AncestorBlock=casper_library_delays/pipeline  mask(pipeline){latency=lat}
      mask help:
      | An explicitly laid-out delay line to avoid mapping to SRL16s
      | for use in pipelining to help achieve timing closure.
      mask init:
      | pipeline_init(gcb,'latency',latency);
      settings: AttributesFormatString=Latency = %<latency>
      mask Display:
      | port_label('input', 1, 'd');
      | port_label('output', 1, 'q');
      | disp(['Z^-', num2str(latency)]);
  pipeline3 : Subsystem  AncestorBlock=casper_library_delays/pipeline  mask(pipeline){latency=lat}
      mask help:
      | An explicitly laid-out delay line to avoid mapping to SRL16s
      | for use in pipelining to help achieve timing closure.
      mask init:
      | pipeline_init(gcb,'latency',latency);
      settings: AttributesFormatString=Latency = %<latency>
      mask Display:
      | port_label('input', 1, 'd');
      | port_label('output', 1, 'q');
      | disp(['Z^-', num2str(latency)]);
  pipeline4 : Subsystem  AncestorBlock=casper_library_delays/pipeline  mask(pipeline){latency=lat}
      mask help:
      | An explicitly laid-out delay line to avoid mapping to SRL16s
      | for use in pipelining to help achieve timing closure.
      mask init:
      | pipeline_init(gcb,'latency',latency);
      settings: AttributesFormatString=Latency = %<latency>
      mask Display:
      | port_label('input', 1, 'd');
      | port_label('output', 1, 'q');
      | disp(['Z^-', num2str(latency)]);
  pipeline5 : Subsystem  AncestorBlock=casper_library_delays/pipeline  mask(pipeline){latency=lat}
      mask help:
      | An explicitly laid-out delay line to avoid mapping to SRL16s
      | for use in pipelining to help achieve timing closure.
      mask init:
      | pipeline_init(gcb,'latency',latency);
      settings: AttributesFormatString=Latency = %<latency>
      mask Display:
      | port_label('input', 1, 'd');
      | port_label('output', 1, 'q');
      | disp(['Z^-', num2str(latency)]);
  pipeline6 : Subsystem  AncestorBlock=casper_library_delays/pipeline  mask(pipeline){latency=lat}
      mask help:
      | An explicitly laid-out delay line to avoid mapping to SRL16s
      | for use in pipelining to help achieve timing closure.
      mask init:
      | pipeline_init(gcb,'latency',latency);
      settings: AttributesFormatString=Latency = %<latency>
      mask Display:
      | port_label('input', 1, 'd');
      | port_label('output', 1, 'q');
      | disp(['Z^-', num2str(latency)]);
  pipeline7 : Subsystem  AncestorBlock=casper_library_delays/pipeline  mask(pipeline){latency=lat}
      mask help:
      | An explicitly laid-out delay line to avoid mapping to SRL16s
      | for use in pipelining to help achieve timing closure.
      mask init:
      | pipeline_init(gcb,'latency',latency);
      settings: AttributesFormatString=Latency = %<latency>
      mask Display:
      | port_label('input', 1, 'd');
      | port_label('output', 1, 'q');
      | disp(['Z^-', num2str(latency)]);
  pipeline8 : Subsystem  AncestorBlock=casper_library_delays/pipeline  mask(pipeline){latency=lat}
      mask help:
      | An explicitly laid-out delay line to avoid mapping to SRL16s
      | for use in pipelining to help achieve timing closure.
      mask init:
      | pipeline_init(gcb,'latency',latency);
      settings: AttributesFormatString=Latency = %<latency>
      mask Display:
      | port_label('input', 1, 'd');
      | port_label('output', 1, 'q');
      | disp(['Z^-', num2str(latency)]);
  pipeline9 : Subsystem  AncestorBlock=casper_library_delays/pipeline  mask(pipeline){latency=lat}
      mask help:
      | An explicitly laid-out delay line to avoid mapping to SRL16s
      | for use in pipelining to help achieve timing closure.
      mask init:
      | pipeline_init(gcb,'latency',latency);
      settings: AttributesFormatString=Latency = %<latency>
      mask Display:
      | port_label('input', 1, 'd');
      | port_label('output', 1, 'q');
      | disp(['Z^-', num2str(latency)]);
  sync_out : Outport
  dou_valid : Outport  Port=2
  pow3_out : Outport  Port=3
  corr3_out : Outport  Port=4
  pow2_out : Outport  Port=5
  corr2_out : Outport  Port=6
  pow1_out : Outport  Port=7
  corr1_out : Outport  Port=8
  pow0_out : Outport  Port=9
  corr0_out : Outport  Port=10
  wires:
  sync_in/1 -> pipeline1/1(d)
  pipeline1/1(q) -> sync_out/1
  din_valid/1 -> pipeline2/1(d)
  pipeline2/1(q) -> dou_valid/1
  pow3_in/1 -> pipeline3/1(d)
  pipeline3/1(q) -> pow3_out/1
  corr3_in/1 -> pipeline4/1(d)
  pipeline4/1(q) -> corr3_out/1
  pow2_in/1 -> pipeline5/1(d)
  pipeline5/1(q) -> pow2_out/1
  corr2_in/1 -> pipeline6/1(d)
  pipeline6/1(q) -> corr2_out/1
  pow1_in/1 -> pipeline7/1(d)
  pipeline7/1(q) -> pow1_out/1
  corr1_in/1 -> pipeline8/1(d)
  pipeline8/1(q) -> corr1_out/1
  pow0_in/1 -> pipeline9/1(d)
  pipeline9/1(q) -> pow0_out/1
  corr0_in/1 -> pipeline10/1(d)
  pipeline10/1(q) -> corr0_out/1

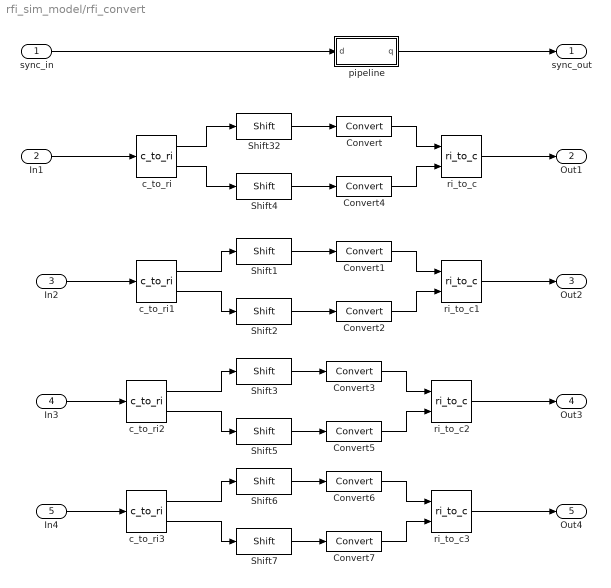
== system rfi_sim_model/rfi_convert ==
  sync_in : Inport
  In1 : Inport  Port=2
  In2 : Inport  Port=3
  In3 : Inport  Port=4
  In4 : Inport  Port=5
  Convert{,1..7} (8 alike) : xbsIndex_r4/Convert  gui_display_data_type=Fixed-point  arith_type="Signed  (2's comp)"  n_bits=conv_width  bin_pt=conv_point  float_type=Single  exp_bits=8  fraction_bits=24  quantization=Truncate  overflow=Wrap  en=off  latency=2  dbl_ovrd=off  pipeline=off  block_type=convert
      settings: block_version=11.4
  Shift{1..7,32} (8 alike) : xbsIndex_r4/Shift  shift_dir=Left  shift_bits=shift_val  en=off  latency=0  precision=Full  arith_type="Signed  (2's comp)"  n_bits=16  bin_pt=14  quantization=Truncate  overflow=Wrap  dbl_ovrd=off  block_type=shift
  c_to_ri{,1..3} (4 alike) : casper_library_misc/c_to_ri  n_bits=18  bin_pt=17
  pipeline : Subsystem  AncestorBlock=casper_library_delays/pipeline  mask(pipeline){latency=2}
      mask help:
      | An explicitly laid-out delay line to avoid mapping to SRL16s
      | for use in pipelining to help achieve timing closure.
      mask init:
      | pipeline_init(gcb,'latency',latency);
      settings: AttributesFormatString=Latency = %<latency>
      mask Display:
      | port_label('input', 1, 'd');
      | port_label('output', 1, 'q');
      | disp(['Z^-', num2str(latency)]);
  ri_to_c{,1..3} (4 alike) : casper_library_misc/ri_to_c
  sync_out : Outport
  Out1 : Outport  Port=2
  Out2 : Outport  Port=3
  Out3 : Outport  Port=4
  Out4 : Outport  Port=5
  wires:
  Shift32/1 -> Convert/1
  sync_in/1 -> pipeline/1(d)
  pipeline/1(q) -> sync_out/1
  In1/1 -> c_to_ri/1
  c_to_ri/1 -> Shift32/1
  ri_to_c/1 -> Out1/1
  Convert/1 -> ri_to_c/1
  Shift4/1 -> Convert4/1
  c_to_ri/2 -> Shift4/1
  Convert4/1 -> ri_to_c/2
  Shift1/1 -> Convert1/1
  c_to_ri1/1 -> Shift1/1
  ri_to_c1/1 -> Out2/1
  Convert1/1 -> ri_to_c1/1
  Shift2/1 -> Convert2/1
  c_to_ri1/2 -> Shift2/1
  Convert2/1 -> ri_to_c1/2
  In2/1 -> c_to_ri1/1
  Shift3/1 -> Convert3/1
  c_to_ri2/1 -> Shift3/1
  ri_to_c2/1 -> Out3/1
  Convert3/1 -> ri_to_c2/1
  Shift5/1 -> Convert5/1
  c_to_ri2/2 -> Shift5/1
  Convert5/1 -> ri_to_c2/2
  In3/1 -> c_to_ri2/1
  Shift6/1 -> Convert6/1
  c_to_ri3/1 -> Shift6/1
  ri_to_c3/1 -> Out4/1
  Convert6/1 -> ri_to_c3/1
  Shift7/1 -> Convert7/1
  c_to_ri3/2 -> Shift7/1
  Convert7/1 -> ri_to_c3/2
  In4/1 -> c_to_ri3/1
